simulink model "ControlloVascaPI_no_du"  (R2022b)
settings: Solver=VariableStepAuto  StartTime=0.0  StopTime=2000  RelTol=1e-3
values from neighbouring files (symbols this model uses):
  Area = 0.08    [ControlloVasca.m]
  Au = 43*1e-6    (= 4.3e-05)    [ControlloVasca.m]
  bx = 0.1    [ControlloVasca.m]
  g = 9.8    [ControlloVasca.m]
  hu = -0.095    [ControlloVasca.m]
  KI = ((-153*0.0027^2))/0.0077    (= -0.144853246753)    [ControlloVasca.m]
  KP = KI/0.0027    (= -53.6493506494)    [ControlloVasca.m]
  L_T = 0:0.01:0.2    [ControlloVasca.m]
  mol = 0.08    [ControlloVasca.m]
  Q_A = 1e-6*[0 8.8 24.6 42.0 57.1 72.4 86.1 102.3 117.6 132.0 144.9]    [ControlloVasca.m]
  rit = 700    [ControlloVasca.m]
  Tn_A = 0:0.5:5    [ControlloVasca.m]
  Tn_T = [4.5221 4.4452 4.2412 3.9653 3.7932 3.5179 3.2742 3.0624 2.8349 2.5936 2.3522 2.1423 1.9151 1.6591 1.4251 1.1892 0.9053 0.7329 0.4750 0.2664 0.0471]    [ControlloVasca.m]
  y0 = 0.1    [ControlloVasca.m]
undefined symbols (not defined in the file or in its folder): A, B, bu, by, C, D
settings Model: Creator=TAWADROS  LastModifiedBy=TAWADROS

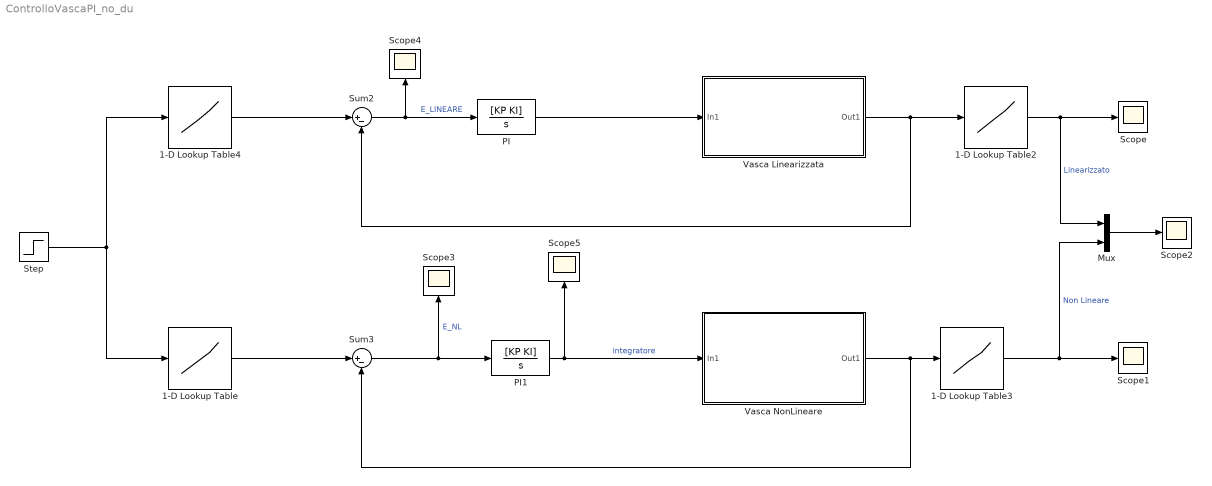
== system ControlloVascaPI_no_du ==
  1-D Lookup Table : Lookup_n-D  NumberOfTableDimensions=1  BreakpointsForDimension1=L_T  Table=Tn_T  InternalRulePriority=Speed  RndMeth=Simplest
  1-D Lookup Table2 : Lookup_n-D  NumberOfTableDimensions=1  BreakpointsForDimension1=fliplr(Tn_T)  Table=fliplr(L_T)  InternalRulePriority=Speed  RndMeth=Simplest
  1-D Lookup Table3 : Lookup_n-D  NumberOfTableDimensions=1  BreakpointsForDimension1=fliplr(Tn_T)  Table=fliplr(L_T)  InternalRulePriority=Speed  RndMeth=Simplest
  1-D Lookup Table4 : Lookup_n-D  NumberOfTableDimensions=1  BreakpointsForDimension1=L_T  Table=Tn_T  InternalRulePriority=Speed  RndMeth=Simplest
  Mux : Mux  Inputs=2
  PI : TransferFcn  Numerator=[KP KI]  Denominator=[1 0]
  PI1 : TransferFcn  Numerator=[KP KI]  Denominator=[1 0]
  Scope{,1..5} (6 alike) : Scope
  Step : Step  Before=y0  After=y0+mol  SampleTime=rit
  Sum2 : Sum  Inputs=|+-
  Sum3 : Sum  Inputs=|+-
  Vasca Linearizzata : Subsystem
  Vasca NonLineare : Subsystem
  wires:
  PI/1 -> Vasca Linearizzata/1(In1)
  Step/1 -> 1-D Lookup Table/1, 1-D Lookup Table4/1
  Sum3/1 -> PI1/1, Scope3/1  "E_NL"
  1-D Lookup Table4/1 -> Sum2/1
  Sum2/1 -> Scope4/1, PI/1  "E_LINEARE"
  1-D Lookup Table/1 -> Sum3/1
  Mux/1 -> Scope2/1
  Vasca Linearizzata/1(Out1) -> 1-D Lookup Table2/1, Sum2/2
  1-D Lookup Table2/1 -> Scope/1, Mux/1  "Linearizzato"
  1-D Lookup Table3/1 -> Mux/2, Scope1/1  "Non Lineare"
  PI1/1 -> Vasca NonLineare/1(In1), Scope5/1  "integratore"
  Vasca NonLineare/1(Out1) -> 1-D Lookup Table3/1, Sum3/2

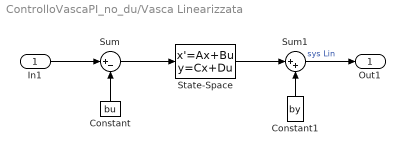
== system ControlloVascaPI_no_du/Vasca Linearizzata ==
  In1 : Inport
  Constant : Constant  Value=bu
  Constant1 : Constant  Value=by
  State-Space : StateSpace  A=A  B=B  C=C  D=D  InitialCondition=0
  Sum : Sum  Inputs=|+-
  Sum1 : Sum  Inputs=|++
  Out1 : Outport
  wires:
  Sum1/1 -> Out1/1  "sys Lin"
  Constant1/1 -> Sum1/2
  Sum/1 -> State-Space/1
  State-Space/1 -> Sum1/1
  In1/1 -> Sum/1
  Constant/1 -> Sum/2

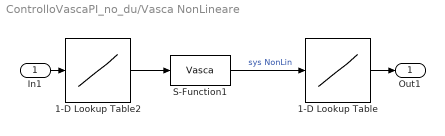
== system ControlloVascaPI_no_du/Vasca NonLineare ==
  In1 : Inport
  1-D Lookup Table : Lookup_n-D  NumberOfTableDimensions=1  BreakpointsForDimension1=L_T  Table=Tn_T  InternalRulePriority=Speed  RndMeth=Simplest
  1-D Lookup Table2 : Lookup_n-D  NumberOfTableDimensions=1  BreakpointsForDimension1=Tn_A  Table=Q_A  InternalRulePriority=Speed  RndMeth=Simplest
  S-Function1 : S-Function  FunctionName=Vasca  Parameters=bx,Area,Au,g,hu  SFunctionDeploymentMode=off  EnableBusSupport=off
  Out1 : Outport
  wires:
  1-D Lookup Table/1 -> Out1/1
  In1/1 -> 1-D Lookup Table2/1
  S-Function1/1 -> 1-D Lookup Table/1  "sys NonLin"
  1-D Lookup Table2/1 -> S-Function1/1
